simulink model "OL_HiLData"  (R2015b)
settings: Solver=FixedStepDiscrete  StartTime=0.0  StopTime=660  FixedStep=step_size  RelTol=1e-3
values from neighbouring files (symbols this model uses):
  step_size = 0.1    [loadCalib.m]
undefined symbols (not defined in the file or in its folder): canChannel, pack_current_eng, pack_current_raw, pack_voltage_eng, pack_voltage_raw, vehicle_voltage_eng, vehicle_voltage_raw
libraries: canmsglib x34, canlib x27, realtime_pacer_lib x1
(part 2 of 2)

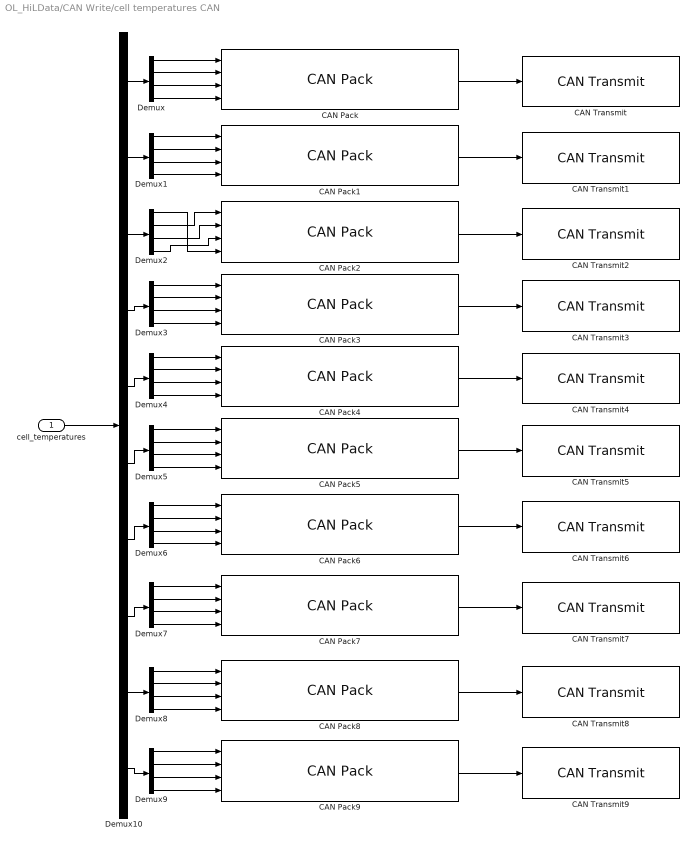
== system OL_HiLData/CAN Write/cell temperatures CAN ==
  cell_temperatures : Inport
  CAN Pack : canmsglib/CAN Pack  CANdbFile=C:\Sagar\Projects\BMS\P006n\08_Work_in_progress\WP3_2_BMS_Stage_1\OpenLoopDataSend\BMSdb.dbc  MsgList=cell_temp_1_4  MsgName=cell_temp_1_4  MsgIDType=Standard (11-bit identifier)  MsgIdentifier=18  MsgLength=8  SignalInfo=cell1_temperature$8$16$2$2$1$0$1.000000e-03$-20$-20$80$#cell2_temperature$24$16$2$2$1$0$1.000000e-03$-20$-20$80$#cell3_temperature$40$16$2$2$1$0$1.000000e-03$-20$-20$80$#cell4_temperature$56$16$2$2$1$0$1.000000e-03$-20$-20$80$#  NSignals=4  StartBits=str2num('[int32(8);int32(24);int32(40);int32(56)]')  SignalSizes=str2num('[int32(16);int32(16);int32(16);int32(16)]')  ByteOrders=str2num('[int32(2);int32(2);int32(2);int32(2)]')  DataTypes=str2num('[int32(2);int32(2);int32(2);int32(2)]')  MultiplexTypes=str2num('[int32(1);int32(1);int32(1);int32(1)]')  MultiplexValues=str2num('[double(0);double(0);double(0);double(0)]')  Factors=str2num('[double(1.000000e-03);double(1.000000e-03);double(1.000000e-03);double(1.000000e-03)]')  Offsets=str2num('[double(-20);double(-20);double(-20);double(-20)]')  Minimums=str2num('[double(-20);double(-20);double(-20);double(-20)]')  Maximums=str2num('[double(80);double(80);double(80);double(80)]')  Remote=off
      settings: DataFormat=CANdb specified signals
  CAN Pack1 : canmsglib/CAN Pack  CANdbFile=C:\Sagar\Projects\BMS\P006n\08_Work_in_progress\WP3_2_BMS_Stage_1\OpenLoopDataSend\BMSdb.dbc  MsgList=cell_temp_5_8  MsgName=cell_temp_5_8  MsgIDType=Standard (11-bit identifier)  MsgIdentifier=19  MsgLength=8  SignalInfo=cell5_temperature$8$16$2$2$1$0$1.000000e-03$-20$-20$80$#cell6_temperature$24$16$2$2$1$0$1.000000e-03$-20$-20$80$#cell7_temperature$40$16$2$2$1$0$1.000000e-03$-20$-20$80$#cell8_temperature$56$16$2$2$1$0$1.000000e-03$-20$-20$80$#  NSignals=4  StartBits=str2num('[int32(8);int32(24);int32(40);int32(56)]')  SignalSizes=str2num('[int32(16);int32(16);int32(16);int32(16)]')  ByteOrders=str2num('[int32(2);int32(2);int32(2);int32(2)]')  DataTypes=str2num('[int32(2);int32(2);int32(2);int32(2)]')  MultiplexTypes=str2num('[int32(1);int32(1);int32(1);int32(1)]')  MultiplexValues=str2num('[double(0);double(0);double(0);double(0)]')  Factors=str2num('[double(1.000000e-03);double(1.000000e-03);double(1.000000e-03);double(1.000000e-03)]')  Offsets=str2num('[double(-20);double(-20);double(-20);double(-20)]')  Minimums=str2num('[double(-20);double(-20);double(-20);double(-20)]')  Maximums=str2num('[double(80);double(80);double(80);double(80)]')  Remote=off
      settings: DataFormat=CANdb specified signals
  CAN Pack2 : canmsglib/CAN Pack  CANdbFile=C:\Sagar\Projects\BMS\P006n\08_Work_in_progress\WP3_2_BMS_Stage_1\OpenLoopDataSend\BMSdb.dbc  MsgList=cell_temp_9_12  MsgName=cell_temp_9_12  MsgIDType=Standard (11-bit identifier)  MsgIdentifier=20  MsgLength=8  SignalInfo=cell10_temperature$24$16$2$2$1$0$1.000000e-03$-20$-20$80$#cell11_temperature$40$16$2$2$1$0$1.000000e-03$-20$-20$80$#cell12_temperature$56$16$2$2$1$0$1.000000e-03$-20$-20$80$#cell9_temperature$8$16$2$2$1$0$1.000000e-03$-20$-20$80$#  NSignals=4  StartBits=str2num('[int32(24);int32(40);int32(56);int32(8)]')  SignalSizes=str2num('[int32(16);int32(16);int32(16);int32(16)]')  ByteOrders=str2num('[int32(2);int32(2);int32(2);int32(2)]')  DataTypes=str2num('[int32(2);int32(2);int32(2);int32(2)]')  MultiplexTypes=str2num('[int32(1);int32(1);int32(1);int32(1)]')  MultiplexValues=str2num('[double(0);double(0);double(0);double(0)]')  Factors=str2num('[double(1.000000e-03);double(1.000000e-03);double(1.000000e-03);double(1.000000e-03)]')  Offsets=str2num('[double(-20);double(-20);double(-20);double(-20)]')  Minimums=str2num('[double(-20);double(-20);double(-20);double(-20)]')  Maximums=str2num('[double(80);double(80);double(80);double(80)]')  Remote=off
      settings: DataFormat=CANdb specified signals
  CAN Pack3 : canmsglib/CAN Pack  CANdbFile=C:\Sagar\Projects\BMS\P006n\08_Work_in_progress\WP3_2_BMS_Stage_1\OpenLoopDataSend\BMSdb.dbc  MsgList=cell_temp_13_16  MsgName=cell_temp_13_16  MsgIDType=Standard (11-bit identifier)  MsgIdentifier=21  MsgLength=8  SignalInfo=cell13_temperature$8$16$2$2$1$0$1.000000e-03$-20$-20$80$#cell14_temperature$24$16$2$2$1$0$1.000000e-03$-20$-20$80$#cell15_temperature$40$16$2$2$1$0$1.000000e-03$-20$-20$80$#cell16_temperature$56$16$2$2$1$0$1.000000e-03$-20$-20$80$#  NSignals=4  StartBits=str2num('[int32(8);int32(24);int32(40);int32(56)]')  SignalSizes=str2num('[int32(16);int32(16);int32(16);int32(16)]')  ByteOrders=str2num('[int32(2);int32(2);int32(2);int32(2)]')  DataTypes=str2num('[int32(2);int32(2);int32(2);int32(2)]')  MultiplexTypes=str2num('[int32(1);int32(1);int32(1);int32(1)]')  MultiplexValues=str2num('[double(0);double(0);double(0);double(0)]')  Factors=str2num('[double(1.000000e-03);double(1.000000e-03);double(1.000000e-03);double(1.000000e-03)]')  Offsets=str2num('[double(-20);double(-20);double(-20);double(-20)]')  Minimums=str2num('[double(-20);double(-20);double(-20);double(-20)]')  Maximums=str2num('[double(80);double(80);double(80);double(80)]')  Remote=off
      settings: DataFormat=CANdb specified signals
  CAN Pack4 : canmsglib/CAN Pack  CANdbFile=C:\Sagar\Projects\BMS\P006n\08_Work_in_progress\WP3_2_BMS_Stage_1\OpenLoopDataSend\BMSdb.dbc  MsgList=cell_temp_17_20  MsgName=cell_temp_17_20  MsgIDType=Standard (11-bit identifier)  MsgIdentifier=22  MsgLength=8  SignalInfo=cell17_temperature$8$16$2$2$1$0$1.000000e-03$-20$-20$80$#cell18_temperature$24$16$2$2$1$0$1.000000e-03$-20$-20$80$#cell19_temperature$40$16$2$2$1$0$1.000000e-03$-20$-20$80$#cell20_temperature$56$16$2$2$1$0$1.000000e-03$-20$-20$80$#  NSignals=4  StartBits=str2num('[int32(8);int32(24);int32(40);int32(56)]')  SignalSizes=str2num('[int32(16);int32(16);int32(16);int32(16)]')  ByteOrders=str2num('[int32(2);int32(2);int32(2);int32(2)]')  DataTypes=str2num('[int32(2);int32(2);int32(2);int32(2)]')  MultiplexTypes=str2num('[int32(1);int32(1);int32(1);int32(1)]')  MultiplexValues=str2num('[double(0);double(0);double(0);double(0)]')  Factors=str2num('[double(1.000000e-03);double(1.000000e-03);double(1.000000e-03);double(1.000000e-03)]')  Offsets=str2num('[double(-20);double(-20);double(-20);double(-20)]')  Minimums=str2num('[double(-20);double(-20);double(-20);double(-20)]')  Maximums=str2num('[double(80);double(80);double(80);double(80)]')  Remote=off
      settings: DataFormat=CANdb specified signals
  CAN Pack5 : canmsglib/CAN Pack  CANdbFile=C:\Sagar\Projects\BMS\P006n\08_Work_in_progress\WP3_2_BMS_Stage_1\OpenLoopDataSend\BMSdb.dbc  MsgList=cell_temp_21_24  MsgName=cell_temp_21_24  MsgIDType=Standard (11-bit identifier)  MsgIdentifier=23  MsgLength=8  SignalInfo=cell21_temperature$8$16$2$2$1$0$1.000000e-03$-20$-20$80$#cell22_temperature$24$16$2$2$1$0$1.000000e-03$-20$-20$80$#cell23_temperature$40$16$2$2$1$0$1.000000e-03$-20$-20$80$#cell24_temperature$56$16$2$2$1$0$1.000000e-03$-20$-20$80$#  NSignals=4  StartBits=str2num('[int32(8);int32(24);int32(40);int32(56)]')  SignalSizes=str2num('[int32(16);int32(16);int32(16);int32(16)]')  ByteOrders=str2num('[int32(2);int32(2);int32(2);int32(2)]')  DataTypes=str2num('[int32(2);int32(2);int32(2);int32(2)]')  MultiplexTypes=str2num('[int32(1);int32(1);int32(1);int32(1)]')  MultiplexValues=str2num('[double(0);double(0);double(0);double(0)]')  Factors=str2num('[double(1.000000e-03);double(1.000000e-03);double(1.000000e-03);double(1.000000e-03)]')  Offsets=str2num('[double(-20);double(-20);double(-20);double(-20)]')  Minimums=str2num('[double(-20);double(-20);double(-20);double(-20)]')  Maximums=str2num('[double(80);double(80);double(80);double(80)]')  Remote=off
      settings: DataFormat=CANdb specified signals
  CAN Pack6 : canmsglib/CAN Pack  CANdbFile=C:\Sagar\Projects\BMS\P006n\08_Work_in_progress\WP3_2_BMS_Stage_1\OpenLoopDataSend\BMSdb.dbc  MsgList=cell_temp_25_28  MsgName=cell_temp_25_28  MsgIDType=Standard (11-bit identifier)  MsgIdentifier=24  MsgLength=8  SignalInfo=cell25_temperature$8$16$2$2$1$0$1.000000e-03$-20$-20$80$#cell26_temperature$24$16$2$2$1$0$1.000000e-03$-20$-20$80$#cell27_temperature$40$16$2$2$1$0$1.000000e-03$-20$-20$80$#cell28_temperature$56$16$2$2$1$0$1.000000e-03$-20$-20$80$#  NSignals=4  StartBits=str2num('[int32(8);int32(24);int32(40);int32(56)]')  SignalSizes=str2num('[int32(16);int32(16);int32(16);int32(16)]')  ByteOrders=str2num('[int32(2);int32(2);int32(2);int32(2)]')  DataTypes=str2num('[int32(2);int32(2);int32(2);int32(2)]')  MultiplexTypes=str2num('[int32(1);int32(1);int32(1);int32(1)]')  MultiplexValues=str2num('[double(0);double(0);double(0);double(0)]')  Factors=str2num('[double(1.000000e-03);double(1.000000e-03);double(1.000000e-03);double(1.000000e-03)]')  Offsets=str2num('[double(-20);double(-20);double(-20);double(-20)]')  Minimums=str2num('[double(-20);double(-20);double(-20);double(-20)]')  Maximums=str2num('[double(80);double(80);double(80);double(80)]')  Remote=off
      settings: DataFormat=CANdb specified signals
  CAN Pack7 : canmsglib/CAN Pack  CANdbFile=C:\Sagar\Projects\BMS\P006n\08_Work_in_progress\WP3_2_BMS_Stage_1\OpenLoopDataSend\BMSdb.dbc  MsgList=cell_temp_29_32  MsgName=cell_temp_29_32  MsgIDType=Standard (11-bit identifier)  MsgIdentifier=25  MsgLength=8  SignalInfo=cell29_temperature$8$16$2$2$1$0$1.000000e-03$-20$-20$80$#cell30_temperature$24$16$2$2$1$0$1.000000e-03$-20$-20$80$#cell31_temperature$40$16$2$2$1$0$1.000000e-03$-20$-20$80$#cell32_temperature$56$16$2$2$1$0$1.000000e-03$-20$-20$80$#  NSignals=4  StartBits=str2num('[int32(8);int32(24);int32(40);int32(56)]')  SignalSizes=str2num('[int32(16);int32(16);int32(16);int32(16)]')  ByteOrders=str2num('[int32(2);int32(2);int32(2);int32(2)]')  DataTypes=str2num('[int32(2);int32(2);int32(2);int32(2)]')  MultiplexTypes=str2num('[int32(1);int32(1);int32(1);int32(1)]')  MultiplexValues=str2num('[double(0);double(0);double(0);double(0)]')  Factors=str2num('[double(1.000000e-03);double(1.000000e-03);double(1.000000e-03);double(1.000000e-03)]')  Offsets=str2num('[double(-20);double(-20);double(-20);double(-20)]')  Minimums=str2num('[double(-20);double(-20);double(-20);double(-20)]')  Maximums=str2num('[double(80);double(80);double(80);double(80)]')  Remote=off
      settings: DataFormat=CANdb specified signals
  CAN Pack8 : canmsglib/CAN Pack  CANdbFile=C:\Sagar\Projects\BMS\P006n\08_Work_in_progress\WP3_2_BMS_Stage_1\OpenLoopDataSend\BMSdb.dbc  MsgList=cell_temp_33_36  MsgName=cell_temp_33_36  MsgIDType=Standard (11-bit identifier)  MsgIdentifier=32  MsgLength=8  SignalInfo=cell33_temperature$8$16$2$2$1$0$1.000000e-03$-20$-20$80$#cell34_temperature$24$16$2$2$1$0$1.000000e-03$-20$-20$80$#cell35_temperature$40$16$2$2$1$0$1.000000e-03$-20$-20$80$#cell36_temperature$56$16$2$2$1$0$1.000000e-03$-20$-20$80$#  NSignals=4  StartBits=str2num('[int32(8);int32(24);int32(40);int32(56)]')  SignalSizes=str2num('[int32(16);int32(16);int32(16);int32(16)]')  ByteOrders=str2num('[int32(2);int32(2);int32(2);int32(2)]')  DataTypes=str2num('[int32(2);int32(2);int32(2);int32(2)]')  MultiplexTypes=str2num('[int32(1);int32(1);int32(1);int32(1)]')  MultiplexValues=str2num('[double(0);double(0);double(0);double(0)]')  Factors=str2num('[double(1.000000e-03);double(1.000000e-03);double(1.000000e-03);double(1.000000e-03)]')  Offsets=str2num('[double(-20);double(-20);double(-20);double(-20)]')  Minimums=str2num('[double(-20);double(-20);double(-20);double(-20)]')  Maximums=str2num('[double(80);double(80);double(80);double(80)]')  Remote=off
      settings: DataFormat=CANdb specified signals
  CAN Pack9 : canmsglib/CAN Pack  CANdbFile=C:\Sagar\Projects\BMS\P006n\08_Work_in_progress\WP3_2_BMS_Stage_1\OpenLoopDataSend\BMSdb.dbc  MsgList=cell_temp_37_40  MsgName=cell_temp_37_40  MsgIDType=Standard (11-bit identifier)  MsgIdentifier=33  MsgLength=8  SignalInfo=cell37_temperature$8$16$2$2$1$0$1.000000e-03$-20$-20$80$#cell38_temperature$24$16$2$2$1$0$1.000000e-03$-20$-20$80$#cell39_temperature$40$16$2$2$1$0$1.000000e-03$-20$-20$80$#cell40_temperature$56$16$2$2$1$0$1.000000e-03$-20$-20$80$#  NSignals=4  StartBits=str2num('[int32(8);int32(24);int32(40);int32(56)]')  SignalSizes=str2num('[int32(16);int32(16);int32(16);int32(16)]')  ByteOrders=str2num('[int32(2);int32(2);int32(2);int32(2)]')  DataTypes=str2num('[int32(2);int32(2);int32(2);int32(2)]')  MultiplexTypes=str2num('[int32(1);int32(1);int32(1);int32(1)]')  MultiplexValues=str2num('[double(0);double(0);double(0);double(0)]')  Factors=str2num('[double(1.000000e-03);double(1.000000e-03);double(1.000000e-03);double(1.000000e-03)]')  Offsets=str2num('[double(-20);double(-20);double(-20);double(-20)]')  Minimums=str2num('[double(-20);double(-20);double(-20);double(-20)]')  Maximums=str2num('[double(80);double(80);double(80);double(80)]')  Remote=off
      settings: DataFormat=CANdb specified signals
  CAN Transmit : canlib/CAN Transmit  BlockHandle=319.0001  DeviceMenu=Kvaser Virtual 1 (Channel 1)  Device=Kvaser USBcan Light 2 (Channel 1)  ObjConstructor=canChannel('Kvaser', 'USBcan Light 2', 1)  EnablePeriodicTransmit=off  MessagePeriod=1.000
  CAN Transmit1 : canlib/CAN Transmit  BlockHandle=320.0001  DeviceMenu=Kvaser Virtual 1 (Channel 1)  Device=Kvaser USBcan Light 2 (Channel 1)  ObjConstructor=canChannel('Kvaser', 'USBcan Light 2', 1)  EnablePeriodicTransmit=off  MessagePeriod=1.000
  CAN Transmit2 : canlib/CAN Transmit  BlockHandle=321.0001  DeviceMenu=Kvaser Virtual 1 (Channel 1)  Device=Kvaser USBcan Light 2 (Channel 1)  ObjConstructor=canChannel('Kvaser', 'USBcan Light 2', 1)  EnablePeriodicTransmit=off  MessagePeriod=1.000
  CAN Transmit3 : canlib/CAN Transmit  BlockHandle=322.0001  DeviceMenu=Kvaser Virtual 1 (Channel 1)  Device=Kvaser USBcan Light 2 (Channel 1)  ObjConstructor=canChannel('Kvaser', 'USBcan Light 2', 1)  EnablePeriodicTransmit=off  MessagePeriod=1.000
  CAN Transmit4 : canlib/CAN Transmit  BlockHandle=323.0001  DeviceMenu=Kvaser Virtual 1 (Channel 1)  Device=Kvaser USBcan Light 2 (Channel 1)  ObjConstructor=canChannel('Kvaser', 'USBcan Light 2', 1)  EnablePeriodicTransmit=off  MessagePeriod=1.000
  CAN Transmit5 : canlib/CAN Transmit  BlockHandle=324.0001  DeviceMenu=Kvaser Virtual 1 (Channel 1)  Device=Kvaser USBcan Light 2 (Channel 1)  ObjConstructor=canChannel('Kvaser', 'USBcan Light 2', 1)  EnablePeriodicTransmit=off  MessagePeriod=1.000
  CAN Transmit6 : canlib/CAN Transmit  BlockHandle=325.0001  DeviceMenu=Kvaser Virtual 1 (Channel 1)  Device=Kvaser USBcan Light 2 (Channel 1)  ObjConstructor=canChannel('Kvaser', 'USBcan Light 2', 1)  EnablePeriodicTransmit=off  MessagePeriod=1.000
  CAN Transmit7 : canlib/CAN Transmit  BlockHandle=326.0001  DeviceMenu=Kvaser Virtual 1 (Channel 1)  Device=Kvaser USBcan Light 2 (Channel 1)  ObjConstructor=canChannel('Kvaser', 'USBcan Light 2', 1)  EnablePeriodicTransmit=off  MessagePeriod=1.000
  CAN Transmit8 : canlib/CAN Transmit  BlockHandle=327.0001  DeviceMenu=Kvaser Virtual 1 (Channel 1)  Device=Kvaser USBcan Light 2 (Channel 1)  ObjConstructor=canChannel('Kvaser', 'USBcan Light 2', 1)  EnablePeriodicTransmit=off  MessagePeriod=1.000
  CAN Transmit9 : canlib/CAN Transmit  BlockHandle=328.0001  DeviceMenu=Kvaser Virtual 1 (Channel 1)  Device=Kvaser USBcan Light 2 (Channel 1)  ObjConstructor=canChannel('Kvaser', 'USBcan Light 2', 1)  EnablePeriodicTransmit=off  MessagePeriod=1.000
  Demux{,1..9} (10 alike) : Demux
  Demux10 : Demux  Outputs=10
  wires:
  Demux5/4 -> CAN Pack5/4
  Demux5/1 -> CAN Pack5/1
  Demux5/2 -> CAN Pack5/2
  Demux5/3 -> CAN Pack5/3
  CAN Pack5/1 -> CAN Transmit5/1
  CAN Pack9/1 -> CAN Transmit9/1
  Demux9/4 -> CAN Pack9/4
  Demux9/1 -> CAN Pack9/1
  Demux9/2 -> CAN Pack9/2
  Demux8/1 -> CAN Pack8/1
  CAN Pack8/1 -> CAN Transmit8/1
  Demux8/3 -> CAN Pack8/3
  Demux8/2 -> CAN Pack8/2
  Demux8/4 -> CAN Pack8/4
  CAN Pack2/1 -> CAN Transmit2/1
  Demux1/4 -> CAN Pack1/4
  CAN Pack1/1 -> CAN Transmit1/1
  Demux1/1 -> CAN Pack1/1
  Demux1/2 -> CAN Pack1/2
  Demux1/3 -> CAN Pack1/3
  Demux4/1 -> CAN Pack4/1
  CAN Pack4/1 -> CAN Transmit4/1
  Demux4/3 -> CAN Pack4/3
  Demux4/2 -> CAN Pack4/2
  Demux4/4 -> CAN Pack4/4
  CAN Pack/1 -> CAN Transmit/1
  Demux/2 -> CAN Pack/2
  Demux/3 -> CAN Pack/3
  Demux/4 -> CAN Pack/4
  Demux6/2 -> CAN Pack6/2
  Demux6/4 -> CAN Pack6/4
  Demux6/3 -> CAN Pack6/3
  CAN Pack6/1 -> CAN Transmit6/1
  Demux6/1 -> CAN Pack6/1
  Demux3/2 -> CAN Pack3/2
  Demux3/1 -> CAN Pack3/1
  CAN Pack3/1 -> CAN Transmit3/1
  Demux3/4 -> CAN Pack3/4
  Demux3/3 -> CAN Pack3/3
  Demux7/2 -> CAN Pack7/2
  Demux7/4 -> CAN Pack7/4
  Demux7/3 -> CAN Pack7/3
  Demux7/1 -> CAN Pack7/1
  CAN Pack7/1 -> CAN Transmit7/1
  Demux10/1 -> Demux/1
  Demux10/2 -> Demux1/1
  Demux10/3 -> Demux2/1
  Demux10/4 -> Demux3/1
  Demux10/5 -> Demux4/1
  Demux10/6 -> Demux5/1
  Demux10/7 -> Demux6/1
  Demux10/8 -> Demux7/1
  Demux10/9 -> Demux8/1
  Demux10/10 -> Demux9/1
  cell_temperatures/1 -> Demux10/1
  Demux/1 -> CAN Pack/1
  Demux9/3 -> CAN Pack9/3
  Demux2/1 -> CAN Pack2/4
  Demux2/2 -> CAN Pack2/1
  Demux2/3 -> CAN Pack2/2
  Demux2/4 -> CAN Pack2/3

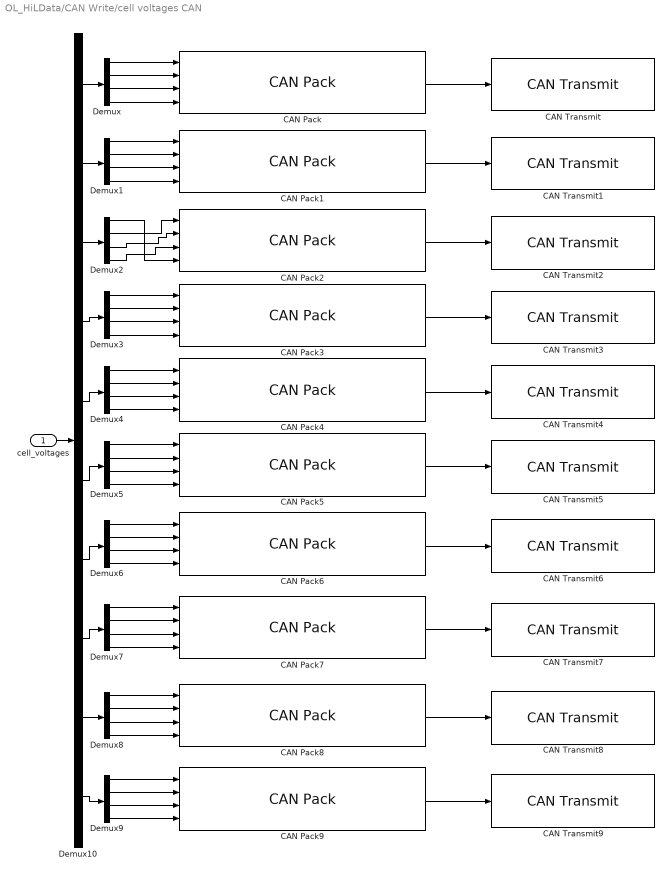
== system OL_HiLData/CAN Write/cell voltages CAN ==
  cell_voltages : Inport
  CAN Pack : canmsglib/CAN Pack  CANdbFile=C:\Sagar\Projects\BMS\P006n\08_Work_in_progress\WP3_2_BMS_Stage_1\OpenLoopDataSend\BMSdb.dbc  MsgList=cell_voltage_1_4  MsgName=cell_voltage_1_4  MsgIDType=Standard (11-bit identifier)  MsgIdentifier=2  MsgLength=8  SignalInfo=cell1_voltage$8$16$2$2$1$0$1.000000e-04$0$0$5$#cell2_voltage$24$16$2$2$1$0$1.000000e-04$0$0$5$#cell3_voltage$40$16$2$2$1$0$1.000000e-04$0$0$5$#cell4_voltage$56$16$2$2$1$0$1.000000e-04$0$0$5$#  NSignals=4  StartBits=str2num('[int32(8);int32(24);int32(40);int32(56)]')  SignalSizes=str2num('[int32(16);int32(16);int32(16);int32(16)]')  ByteOrders=str2num('[int32(2);int32(2);int32(2);int32(2)]')  DataTypes=str2num('[int32(2);int32(2);int32(2);int32(2)]')  MultiplexTypes=str2num('[int32(1);int32(1);int32(1);int32(1)]')  MultiplexValues=str2num('[double(0);double(0);double(0);double(0)]')  Factors=str2num('[double(1.000000e-04);double(1.000000e-04);double(1.000000e-04);double(1.000000e-04)]')  Offsets=str2num('[double(0);double(0);double(0);double(0)]')  Minimums=str2num('[double(0);double(0);double(0);double(0)]')  Maximums=str2num('[double(5);double(5);double(5);double(5)]')  Remote=off
      settings: DataFormat=CANdb specified signals
  CAN Pack1 : canmsglib/CAN Pack  CANdbFile=C:\Sagar\Projects\BMS\P006n\08_Work_in_progress\WP3_2_BMS_Stage_1\OpenLoopDataSend\BMSdb.dbc  MsgList=cell_voltage_5_8  MsgName=cell_voltage_5_8  MsgIDType=Standard (11-bit identifier)  MsgIdentifier=3  MsgLength=8  SignalInfo=cell5_votlage$8$16$2$2$1$0$1.000000e-04$0$0$5$#cell6_voltage$24$16$2$2$1$0$1.000000e-04$0$0$5$#cell7_voltage$40$16$2$2$1$0$1.000000e-04$0$0$5$#cell8_voltage$56$16$2$2$1$0$1.000000e-04$0$0$5$#  NSignals=4  StartBits=str2num('[int32(8);int32(24);int32(40);int32(56)]')  SignalSizes=str2num('[int32(16);int32(16);int32(16);int32(16)]')  ByteOrders=str2num('[int32(2);int32(2);int32(2);int32(2)]')  DataTypes=str2num('[int32(2);int32(2);int32(2);int32(2)]')  MultiplexTypes=str2num('[int32(1);int32(1);int32(1);int32(1)]')  MultiplexValues=str2num('[double(0);double(0);double(0);double(0)]')  Factors=str2num('[double(1.000000e-04);double(1.000000e-04);double(1.000000e-04);double(1.000000e-04)]')  Offsets=str2num('[double(0);double(0);double(0);double(0)]')  Minimums=str2num('[double(0);double(0);double(0);double(0)]')  Maximums=str2num('[double(5);double(5);double(5);double(5)]')  Remote=off
      settings: DataFormat=CANdb specified signals
  CAN Pack2 : canmsglib/CAN Pack  CANdbFile=C:\Sagar\Projects\BMS\P006n\08_Work_in_progress\WP3_2_BMS_Stage_1\OpenLoopDataSend\BMSdb.dbc  MsgList=cell_voltage_9_12  MsgName=cell_voltage_9_12  MsgIDType=Standard (11-bit identifier)  MsgIdentifier=4  MsgLength=8  SignalInfo=cell10_voltage$24$16$2$2$1$0$1.000000e-04$0$0$5$#cell11_voltage$40$16$2$2$1$0$1.000000e-04$0$0$5$#cell12_voltage$56$16$2$2$1$0$1.000000e-04$0$0$5$#cell9_votlage$8$16$2$2$1$0$1.000000e-04$0$0$5$#  NSignals=4  StartBits=str2num('[int32(24);int32(40);int32(56);int32(8)]')  SignalSizes=str2num('[int32(16);int32(16);int32(16);int32(16)]')  ByteOrders=str2num('[int32(2);int32(2);int32(2);int32(2)]')  DataTypes=str2num('[int32(2);int32(2);int32(2);int32(2)]')  MultiplexTypes=str2num('[int32(1);int32(1);int32(1);int32(1)]')  MultiplexValues=str2num('[double(0);double(0);double(0);double(0)]')  Factors=str2num('[double(1.000000e-04);double(1.000000e-04);double(1.000000e-04);double(1.000000e-04)]')  Offsets=str2num('[double(0);double(0);double(0);double(0)]')  Minimums=str2num('[double(0);double(0);double(0);double(0)]')  Maximums=str2num('[double(5);double(5);double(5);double(5)]')  Remote=off
      settings: DataFormat=CANdb specified signals
  CAN Pack3 : canmsglib/CAN Pack  CANdbFile=C:\Sagar\Projects\BMS\P006n\08_Work_in_progress\WP3_2_BMS_Stage_1\OpenLoopDataSend\BMSdb.dbc  MsgList=cell_voltage_13_16  MsgName=cell_voltage_13_16  MsgIDType=Standard (11-bit identifier)  MsgIdentifier=5  MsgLength=8  SignalInfo=cell13_votlage$8$16$2$2$1$0$1.000000e-04$0$0$5$#cell14_voltage$24$16$2$2$1$0$1.000000e-04$0$0$5$#cell15_voltage$40$16$2$2$1$0$1.000000e-04$0$0$5$#cell16_voltage$56$16$2$2$1$0$1.000000e-04$0$0$5$#  NSignals=4  StartBits=str2num('[int32(8);int32(24);int32(40);int32(56)]')  SignalSizes=str2num('[int32(16);int32(16);int32(16);int32(16)]')  ByteOrders=str2num('[int32(2);int32(2);int32(2);int32(2)]')  DataTypes=str2num('[int32(2);int32(2);int32(2);int32(2)]')  MultiplexTypes=str2num('[int32(1);int32(1);int32(1);int32(1)]')  MultiplexValues=str2num('[double(0);double(0);double(0);double(0)]')  Factors=str2num('[double(1.000000e-04);double(1.000000e-04);double(1.000000e-04);double(1.000000e-04)]')  Offsets=str2num('[double(0);double(0);double(0);double(0)]')  Minimums=str2num('[double(0);double(0);double(0);double(0)]')  Maximums=str2num('[double(5);double(5);double(5);double(5)]')  Remote=off
      settings: DataFormat=CANdb specified signals
  CAN Pack4 : canmsglib/CAN Pack  CANdbFile=C:\Sagar\Projects\BMS\P006n\08_Work_in_progress\WP3_2_BMS_Stage_1\OpenLoopDataSend\BMSdb.dbc  MsgList=cell_voltage_17_20  MsgName=cell_voltage_17_20  MsgIDType=Standard (11-bit identifier)  MsgIdentifier=6  MsgLength=8  SignalInfo=cell17_votlage$8$16$2$2$1$0$1.000000e-04$0$0$5$#cell18_voltage$24$16$2$2$1$0$1.000000e-04$0$0$5$#cell19_voltage$40$16$2$2$1$0$1.000000e-04$0$0$5$#cell20_voltage$56$16$2$2$1$0$1.000000e-04$0$0$5$#  NSignals=4  StartBits=str2num('[int32(8);int32(24);int32(40);int32(56)]')  SignalSizes=str2num('[int32(16);int32(16);int32(16);int32(16)]')  ByteOrders=str2num('[int32(2);int32(2);int32(2);int32(2)]')  DataTypes=str2num('[int32(2);int32(2);int32(2);int32(2)]')  MultiplexTypes=str2num('[int32(1);int32(1);int32(1);int32(1)]')  MultiplexValues=str2num('[double(0);double(0);double(0);double(0)]')  Factors=str2num('[double(1.000000e-04);double(1.000000e-04);double(1.000000e-04);double(1.000000e-04)]')  Offsets=str2num('[double(0);double(0);double(0);double(0)]')  Minimums=str2num('[double(0);double(0);double(0);double(0)]')  Maximums=str2num('[double(5);double(5);double(5);double(5)]')  Remote=off
      settings: DataFormat=CANdb specified signals
  CAN Pack5 : canmsglib/CAN Pack  CANdbFile=C:\Sagar\Projects\BMS\P006n\08_Work_in_progress\WP3_2_BMS_Stage_1\OpenLoopDataSend\BMSdb.dbc  MsgList=cell_voltage_21_24  MsgName=cell_voltage_21_24  MsgIDType=Standard (11-bit identifier)  MsgIdentifier=7  MsgLength=8  SignalInfo=cell21_votlage$8$16$2$2$1$0$1.000000e-04$0$0$5$#cell22_votlage$24$16$2$2$1$0$1.000000e-04$0$0$5$#cell23_votlage$40$16$2$2$1$0$1.000000e-04$0$0$5$#cell24_votlage$56$16$2$2$1$0$1.000000e-04$0$0$5$#  NSignals=4  StartBits=str2num('[int32(8);int32(24);int32(40);int32(56)]')  SignalSizes=str2num('[int32(16);int32(16);int32(16);int32(16)]')  ByteOrders=str2num('[int32(2);int32(2);int32(2);int32(2)]')  DataTypes=str2num('[int32(2);int32(2);int32(2);int32(2)]')  MultiplexTypes=str2num('[int32(1);int32(1);int32(1);int32(1)]')  MultiplexValues=str2num('[double(0);double(0);double(0);double(0)]')  Factors=str2num('[double(1.000000e-04);double(1.000000e-04);double(1.000000e-04);double(1.000000e-04)]')  Offsets=str2num('[double(0);double(0);double(0);double(0)]')  Minimums=str2num('[double(0);double(0);double(0);double(0)]')  Maximums=str2num('[double(5);double(5);double(5);double(5)]')  Remote=off
      settings: DataFormat=CANdb specified signals
  CAN Pack6 : canmsglib/CAN Pack  CANdbFile=C:\Sagar\Projects\BMS\P006n\08_Work_in_progress\WP3_2_BMS_Stage_1\OpenLoopDataSend\BMSdb.dbc  MsgList=cell_voltage_25_28  MsgName=cell_voltage_25_28  MsgIDType=Standard (11-bit identifier)  MsgIdentifier=8  MsgLength=8  SignalInfo=cell25_votlage$8$16$2$2$1$0$1.000000e-04$0$0$5$#cell26_votlage$24$16$2$2$1$0$1.000000e-04$0$0$5$#cell27_votlage$40$16$2$2$1$0$1.000000e-04$0$0$5$#cell28_votlage$56$16$2$2$1$0$1.000000e-04$0$0$5$#  NSignals=4  StartBits=str2num('[int32(8);int32(24);int32(40);int32(56)]')  SignalSizes=str2num('[int32(16);int32(16);int32(16);int32(16)]')  ByteOrders=str2num('[int32(2);int32(2);int32(2);int32(2)]')  DataTypes=str2num('[int32(2);int32(2);int32(2);int32(2)]')  MultiplexTypes=str2num('[int32(1);int32(1);int32(1);int32(1)]')  MultiplexValues=str2num('[double(0);double(0);double(0);double(0)]')  Factors=str2num('[double(1.000000e-04);double(1.000000e-04);double(1.000000e-04);double(1.000000e-04)]')  Offsets=str2num('[double(0);double(0);double(0);double(0)]')  Minimums=str2num('[double(0);double(0);double(0);double(0)]')  Maximums=str2num('[double(5);double(5);double(5);double(5)]')  Remote=off
      settings: DataFormat=CANdb specified signals
  CAN Pack7 : canmsglib/CAN Pack  CANdbFile=C:\Sagar\Projects\BMS\P006n\08_Work_in_progress\WP3_2_BMS_Stage_1\OpenLoopDataSend\BMSdb.dbc  MsgList=cell_voltage_29_32  MsgName=cell_voltage_29_32  MsgIDType=Standard (11-bit identifier)  MsgIdentifier=9  MsgLength=8  SignalInfo=cell29_votlage$8$16$2$2$1$0$1.000000e-04$0$0$5$#cell30_votlage$24$16$2$2$1$0$1.000000e-04$0$0$5$#cell31_votlage$40$16$2$2$1$0$1.000000e-04$0$0$5$#cell32_votlage$56$16$2$2$1$0$1.000000e-04$0$0$5$#  NSignals=4  StartBits=str2num('[int32(8);int32(24);int32(40);int32(56)]')  SignalSizes=str2num('[int32(16);int32(16);int32(16);int32(16)]')  ByteOrders=str2num('[int32(2);int32(2);int32(2);int32(2)]')  DataTypes=str2num('[int32(2);int32(2);int32(2);int32(2)]')  MultiplexTypes=str2num('[int32(1);int32(1);int32(1);int32(1)]')  MultiplexValues=str2num('[double(0);double(0);double(0);double(0)]')  Factors=str2num('[double(1.000000e-04);double(1.000000e-04);double(1.000000e-04);double(1.000000e-04)]')  Offsets=str2num('[double(0);double(0);double(0);double(0)]')  Minimums=str2num('[double(0);double(0);double(0);double(0)]')  Maximums=str2num('[double(5);double(5);double(5);double(5)]')  Remote=off
      settings: DataFormat=CANdb specified signals
  CAN Pack8 : canmsglib/CAN Pack  CANdbFile=C:\Sagar\Projects\BMS\P006n\08_Work_in_progress\WP3_2_BMS_Stage_1\OpenLoopDataSend\BMSdb.dbc  MsgList=cell_voltage_33_36  MsgName=cell_voltage_33_36  MsgIDType=Standard (11-bit identifier)  MsgIdentifier=16  MsgLength=8  SignalInfo=cell33_votlage$8$16$2$2$1$0$1.000000e-04$0$0$5$#cell34_votlage$24$16$2$2$1$0$1.000000e-04$0$0$5$#cell35_votlage$40$16$2$2$1$0$1.000000e-04$0$0$5$#cell36_votlage$56$16$2$2$1$0$1.000000e-04$0$0$5$#  NSignals=4  StartBits=str2num('[int32(8);int32(24);int32(40);int32(56)]')  SignalSizes=str2num('[int32(16);int32(16);int32(16);int32(16)]')  ByteOrders=str2num('[int32(2);int32(2);int32(2);int32(2)]')  DataTypes=str2num('[int32(2);int32(2);int32(2);int32(2)]')  MultiplexTypes=str2num('[int32(1);int32(1);int32(1);int32(1)]')  MultiplexValues=str2num('[double(0);double(0);double(0);double(0)]')  Factors=str2num('[double(1.000000e-04);double(1.000000e-04);double(1.000000e-04);double(1.000000e-04)]')  Offsets=str2num('[double(0);double(0);double(0);double(0)]')  Minimums=str2num('[double(0);double(0);double(0);double(0)]')  Maximums=str2num('[double(5);double(5);double(5);double(5)]')  Remote=off
      settings: DataFormat=CANdb specified signals
  CAN Pack9 : canmsglib/CAN Pack  CANdbFile=C:\Sagar\Projects\BMS\P006n\08_Work_in_progress\WP3_2_BMS_Stage_1\OpenLoopDataSend\BMSdb.dbc  MsgList=cell_voltage_37_40  MsgName=cell_voltage_37_40  MsgIDType=Standard (11-bit identifier)  MsgIdentifier=17  MsgLength=8  SignalInfo=cell37_votlage$8$16$2$2$1$0$1.000000e-04$0$0$5$#cell38_votlage$24$16$2$2$1$0$1.000000e-04$0$0$5$#cell39_votlage$40$16$2$2$1$0$1.000000e-04$0$0$5$#cell40_votlage$56$16$2$2$1$0$1.000000e-04$0$0$5$#  NSignals=4  StartBits=str2num('[int32(8);int32(24);int32(40);int32(56)]')  SignalSizes=str2num('[int32(16);int32(16);int32(16);int32(16)]')  ByteOrders=str2num('[int32(2);int32(2);int32(2);int32(2)]')  DataTypes=str2num('[int32(2);int32(2);int32(2);int32(2)]')  MultiplexTypes=str2num('[int32(1);int32(1);int32(1);int32(1)]')  MultiplexValues=str2num('[double(0);double(0);double(0);double(0)]')  Factors=str2num('[double(1.000000e-04);double(1.000000e-04);double(1.000000e-04);double(1.000000e-04)]')  Offsets=str2num('[double(0);double(0);double(0);double(0)]')  Minimums=str2num('[double(0);double(0);double(0);double(0)]')  Maximums=str2num('[double(5);double(5);double(5);double(5)]')  Remote=off
      settings: DataFormat=CANdb specified signals
  CAN Transmit : canlib/CAN Transmit  BlockHandle=413.0001  DeviceMenu=Kvaser Virtual 1 (Channel 1)  Device=Kvaser USBcan Light 2 (Channel 1)  ObjConstructor=canChannel('Kvaser', 'USBcan Light 2', 1)  EnablePeriodicTransmit=off  MessagePeriod=1.000
  CAN Transmit1 : canlib/CAN Transmit  BlockHandle=414.0001  DeviceMenu=Kvaser Virtual 1 (Channel 1)  Device=Kvaser USBcan Light 2 (Channel 1)  ObjConstructor=canChannel('Kvaser', 'USBcan Light 2', 1)  EnablePeriodicTransmit=off  MessagePeriod=1.000
  CAN Transmit2 : canlib/CAN Transmit  BlockHandle=415.0001  DeviceMenu=Kvaser Virtual 1 (Channel 1)  Device=Kvaser USBcan Light 2 (Channel 1)  ObjConstructor=canChannel('Kvaser', 'USBcan Light 2', 1)  EnablePeriodicTransmit=off  MessagePeriod=1.000
  CAN Transmit3 : canlib/CAN Transmit  BlockHandle=416.0001  DeviceMenu=Kvaser Virtual 1 (Channel 1)  Device=Kvaser USBcan Light 2 (Channel 1)  ObjConstructor=canChannel('Kvaser', 'USBcan Light 2', 1)  EnablePeriodicTransmit=off  MessagePeriod=1.000
  CAN Transmit4 : canlib/CAN Transmit  BlockHandle=417.0001  DeviceMenu=Kvaser Virtual 1 (Channel 1)  Device=Kvaser USBcan Light 2 (Channel 1)  ObjConstructor=canChannel('Kvaser', 'USBcan Light 2', 1)  EnablePeriodicTransmit=off  MessagePeriod=1.000
  CAN Transmit5 : canlib/CAN Transmit  BlockHandle=418.0001  DeviceMenu=Kvaser Virtual 1 (Channel 1)  Device=Kvaser USBcan Light 2 (Channel 1)  ObjConstructor=canChannel('Kvaser', 'USBcan Light 2', 1)  EnablePeriodicTransmit=off  MessagePeriod=1.000
  CAN Transmit6 : canlib/CAN Transmit  BlockHandle=419.0001  DeviceMenu=Kvaser Virtual 1 (Channel 1)  Device=Kvaser USBcan Light 2 (Channel 1)  ObjConstructor=canChannel('Kvaser', 'USBcan Light 2', 1)  EnablePeriodicTransmit=off  MessagePeriod=1.000
  CAN Transmit7 : canlib/CAN Transmit  BlockHandle=420.0001  DeviceMenu=Kvaser Virtual 1 (Channel 1)  Device=Kvaser USBcan Light 2 (Channel 1)  ObjConstructor=canChannel('Kvaser', 'USBcan Light 2', 1)  EnablePeriodicTransmit=off  MessagePeriod=1.000
  CAN Transmit8 : canlib/CAN Transmit  BlockHandle=421.0001  DeviceMenu=Kvaser Virtual 1 (Channel 1)  Device=Kvaser USBcan Light 2 (Channel 1)  ObjConstructor=canChannel('Kvaser', 'USBcan Light 2', 1)  EnablePeriodicTransmit=off  MessagePeriod=1.000
  CAN Transmit9 : canlib/CAN Transmit  BlockHandle=422.0001  DeviceMenu=Kvaser Virtual 1 (Channel 1)  Device=Kvaser USBcan Light 2 (Channel 1)  ObjConstructor=canChannel('Kvaser', 'USBcan Light 2', 1)  EnablePeriodicTransmit=off  MessagePeriod=1.000
  Demux{,1..9} (10 alike) : Demux
  Demux10 : Demux  Outputs=10
  wires:
  Demux5/4 -> CAN Pack5/4
  Demux5/1 -> CAN Pack5/1
  Demux5/2 -> CAN Pack5/2
  Demux5/3 -> CAN Pack5/3
  CAN Pack5/1 -> CAN Transmit5/1
  CAN Pack9/1 -> CAN Transmit9/1
  Demux9/4 -> CAN Pack9/4
  Demux9/1 -> CAN Pack9/1
  Demux9/2 -> CAN Pack9/2
  Demux8/1 -> CAN Pack8/1
  CAN Pack8/1 -> CAN Transmit8/1
  Demux8/3 -> CAN Pack8/3
  Demux8/2 -> CAN Pack8/2
  Demux8/4 -> CAN Pack8/4
  CAN Pack2/1 -> CAN Transmit2/1
  Demux1/4 -> CAN Pack1/4
  CAN Pack1/1 -> CAN Transmit1/1
  Demux1/1 -> CAN Pack1/1
  Demux1/2 -> CAN Pack1/2
  Demux1/3 -> CAN Pack1/3
  Demux4/1 -> CAN Pack4/1
  CAN Pack4/1 -> CAN Transmit4/1
  Demux4/3 -> CAN Pack4/3
  Demux4/2 -> CAN Pack4/2
  Demux4/4 -> CAN Pack4/4
  CAN Pack/1 -> CAN Transmit/1
  Demux/2 -> CAN Pack/2
  Demux/3 -> CAN Pack/3
  Demux/4 -> CAN Pack/4
  Demux6/2 -> CAN Pack6/2
  Demux6/4 -> CAN Pack6/4
  Demux6/3 -> CAN Pack6/3
  CAN Pack6/1 -> CAN Transmit6/1
  Demux6/1 -> CAN Pack6/1
  Demux3/2 -> CAN Pack3/2
  Demux3/1 -> CAN Pack3/1
  CAN Pack3/1 -> CAN Transmit3/1
  Demux3/4 -> CAN Pack3/4
  Demux3/3 -> CAN Pack3/3
  Demux7/2 -> CAN Pack7/2
  Demux7/4 -> CAN Pack7/4
  Demux7/3 -> CAN Pack7/3
  Demux7/1 -> CAN Pack7/1
  CAN Pack7/1 -> CAN Transmit7/1
  Demux10/1 -> Demux/1
  Demux10/2 -> Demux1/1
  Demux10/3 -> Demux2/1
  Demux10/4 -> Demux3/1
  Demux10/5 -> Demux4/1
  Demux10/6 -> Demux5/1
  Demux10/7 -> Demux6/1
  Demux10/8 -> Demux7/1
  Demux10/9 -> Demux8/1
  Demux10/10 -> Demux9/1
  cell_voltages/1 -> Demux10/1
  Demux/1 -> CAN Pack/1
  Demux9/3 -> CAN Pack9/3
  Demux2/1 -> CAN Pack2/4
  Demux2/2 -> CAN Pack2/1
  Demux2/3 -> CAN Pack2/2
  Demux2/4 -> CAN Pack2/3

== matlab function OL_HiLData/Analog Outputs Labjack1/MATLAB Function3 ==
  data: DAC0state_packVoltage input; DAC1state_vehicleVoltage input
function publishAnalogOut(DAC0state_packVoltage, DAC1state_vehicleVoltage)

pubstates = [DAC0state_packVoltage, DAC1state_vehicleVoltage];
pins = {'DAC0','DAC1'};
sno = '440012786';
coder.extrinsic('writeOut');
writeOut(pubstates,pins,sno);

end

== matlab function OL_HiLData/Analog Outputs Labjack2/MATLAB Function3 ==
  data: DAC0state_packCurrent input; DAC1state_hvilReturn input
function publishAnalogOut(DAC0state_packCurrent, DAC1state_hvilReturn)

pubstates = [DAC0state_packCurrent,DAC1state_hvilReturn];
pins = {'DAC0','DAC1'};
sno = '440012853';
coder.extrinsic('writeOut');
writeOut(pubstates,pins,sno);
 
end

== matlab function OL_HiLData/Digital Inputs Labjack2/MATLAB Function2 ==
  data: main_cc_cmd output; pre_chg_cc_cmd output; neg_cc_cmd output; cvtn_wake_up output
function [main_cc_cmd, pre_chg_cc_cmd, neg_cc_cmd, cvtn_wake_up] = readDigitalInput()

out = zeros(1,4);

pins = {'FIO4','FIO5','FIO6','FIO7'};
sno = '440012853';
coder.extrinsic('readIn');
out = readIn(pins,sno);

main_cc_cmd = out(1);
pre_chg_cc_cmd = out(2);
neg_cc_cmd = out(3);
cvtn_wake_up = out(4);

end

== matlab function OL_HiLData/Digital Outputs Labjack1/MATLAB Function3 ==
  data: FIO4state_key input
function publishDigitalOut(FIO4state_key)

pubstates = [FIO4state_key];
pins = {'FIO4'};
sno = '440012786';
coder.extrinsic('writeOut');
writeOut(pubstates,pins,sno);

end

== matlab function OL_HiLData/Analog Inputs Labjack1/MATLAB Function2 ==
  data: fan_cmd output
function fan_cmd  = readAnalogInput

out = zeros(1,1);

pins = {'AIN0'};
sno = '440012786';
coder.extrinsic('readIn');
out = readIn(pins,sno);

fan_cmd = out(1);

end
